simulink model "elektricnimodel"  (R2017b)
settings: Solver=ode15s  StartTime=0.0  StopTime=10.0  RelTol=1e-3
values from neighbouring files (symbols this model uses):
  otpor = str2num(get(handles.otpor,'String'))    [gui.m]
libraries: fl_lib x6, nesl_utility x4, elec_lib x2
settings Model: Creator=USER  LastModifiedBy=USER

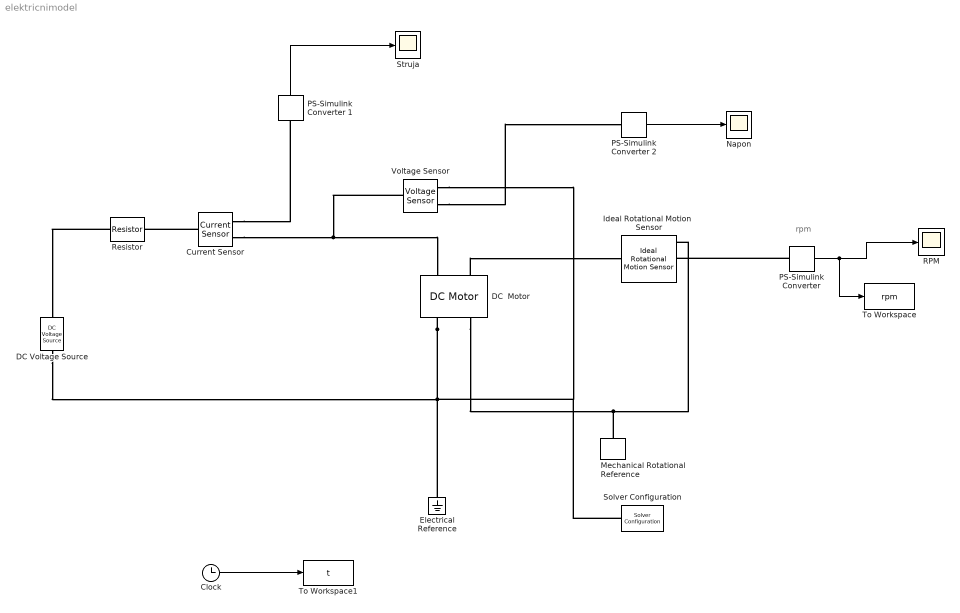
== system elektricnimodel ==
  note: rpm
  Clock : Clock
  "Current Sensor " : fl_lib/Electrical/Electrical Sensors/Current Sensor
  DC  Motor : elec_lib/Actuators & Drivers/Rotational Actuators/DC Motor  parameterization=1  Ra=3.9 Ohm  La=12e-5 H  emf_or_torque=1  Kv=7.2e-5 V/rpm  Ki=6.876e-4 N*m/A  T_stall=0.24e-3 N*m  w_max=19100 rpm  w_rated=15000 rpm  P_rated=0.08 W  V_rated=1.5 V  J=0.01 g*cm^2  lam_param=1  lam=0.000000001 N*m/(rad/s)  i_noload=0 A  V_i_noload=1.5 V  speed0=0 rpm  alpha=3.93e-3 1/K  Tmeas=25 degC  thermal_mass=100 J/K  initial_temperature=25 degC
  "DC Voltage Source " : elec_lib/Additional Components/SPICE-Compatible Components/Sources/DC Voltage Source  DC=12 V
      settings: SourceProductName=Simscape Electronics  SourceProductBaseCode=SN
  "Electrical Reference " : fl_lib/Electrical/Electrical Elements/Electrical Reference
  Ideal Rotational Motion  Sensor : fl_lib/Mechanical/Mechanical Sensors/Ideal Rotational Motion Sensor  offset=0 rad
  Mechanical Rotational Reference : fl_lib/Mechanical/Rotational Elements/Mechanical Rotational Reference
  Napon : Scope
  "PS-Simulink Converter " : nesl_utility/PS-Simulink Converter  PhysicalDomain=network_engine_domain  SubClassName=ps_output  LeftPortType=input  RightPortType=output  PseudoPeriodic=off  Frequencies=[]  Unit=rpm  AffineConversion=off
  PS-Simulink Converter 1 : nesl_utility/PS-Simulink Converter  PhysicalDomain=network_engine_domain  SubClassName=ps_output  LeftPortType=input  RightPortType=output  PseudoPeriodic=off  Frequencies=[]  Unit=A  AffineConversion=off
  PS-Simulink Converter 2 : nesl_utility/PS-Simulink Converter  PhysicalDomain=network_engine_domain  SubClassName=ps_output  LeftPortType=input  RightPortType=output  PseudoPeriodic=off  Frequencies=[]  Unit=V  AffineConversion=off
  RPM : Scope
  Resistor : fl_lib/Electrical/Electrical Elements/Resistor  R=otpor Ohm  i_specify=off  i_priority=None  i=0 A  i_nominal_specify=off  i_nominal_unit=A  i_nominal_value=1  v_specify=off  v_priority=None  v=0 V  v_nominal_specify=off  v_nominal_unit=V  v_nominal_value=1
  "Solver Configuration " : nesl_utility/Solver Configuration  PhysicalDomain=network_engine_domain  SubClassName=solver  LeftPortType=input  RightPortType=generic  Accelerate=off  Tones=[]  Harmonics=[]  SimulateNoise=off  Profile=off  UseLocalSampling=off  EnableSwitchedLinearOptims=on  FrequencyDomain=off  UseCCode=off  RelTol=0.001  AbsTol=1e-06  MinStep=1e-09  ToWorkspace=off  RevertToSquareIcSolve=off  NumHomotopyIterations=100  PhasorMode=off  PhasorModeNumHarmonics=1  DoDC=off  ResidualTolerance=1e-09  UseLocalSolver=off  LocalSolverChoice=NE_BACKWARD_EULER_ADVANCER  LocalSolverSampleTime=0.001  DoFixedCost=off  MaxNonlinIter=3  MaxModeIter=2  LinearAlgebra=Sparse  DelaysMemoryBudget=1024  AutomaticFiltering=on  FilteringTimeConstant=0.001
  Struja : Scope
  "To Workspace " : ToWorkspace  VariableName=rpm  SampleTime=-1
  To Workspace1 : ToWorkspace  VariableName=t  SampleTime=-1
  "Voltage Sensor " : fl_lib/Electrical/Electrical Sensors/Voltage Sensor
  wires:
  PS-Simulink Converter 2/1 -> Napon/1
  PS-Simulink Converter 1/1 -> Struja/1
  Clock/1 -> To Workspace1/1
  "PS-Simulink Converter "/1 -> "To Workspace "/1, RPM/1
  connections:
  DC  Motor/RConn2 -- Mechanical Rotational Reference/LConn1 -- Ideal Rotational Motion  Sensor/RConn1
  "Current Sensor "/RConn2 -- "Voltage Sensor "/LConn1 -- DC  Motor/LConn1
  DC  Motor/RConn1 -- "Solver Configuration "/RConn1 -- "Voltage Sensor "/RConn2 -- "DC Voltage Source "/RConn1 -- "Electrical Reference "/LConn1
  "Current Sensor "/RConn1 -- PS-Simulink Converter 1/LConn1
  "Current Sensor "/LConn1 -- Resistor/RConn1
  "Voltage Sensor "/RConn1 -- PS-Simulink Converter 2/LConn1
  "PS-Simulink Converter "/LConn1 -- Ideal Rotational Motion  Sensor/RConn2
  Resistor/LConn1 -- "DC Voltage Source "/LConn1
  DC  Motor/LConn2 -- Ideal Rotational Motion  Sensor/LConn1
